simulink model "duffingSystem"  (R2020b)
settings: Solver=VariableStepAuto  StartTime=0.0  StopTime=60  RelTol=1e-8
values from neighbouring files (symbols this model uses):
  flag = 1    [aae666_hw4_p4.m]
  k1 = 1.25    [aae666_hw4_p4.m]
  k2 = 1.5    [aae666_hw4_p4.m]
settings Model: Creator=Tomo  LastModifiedBy=Tomo

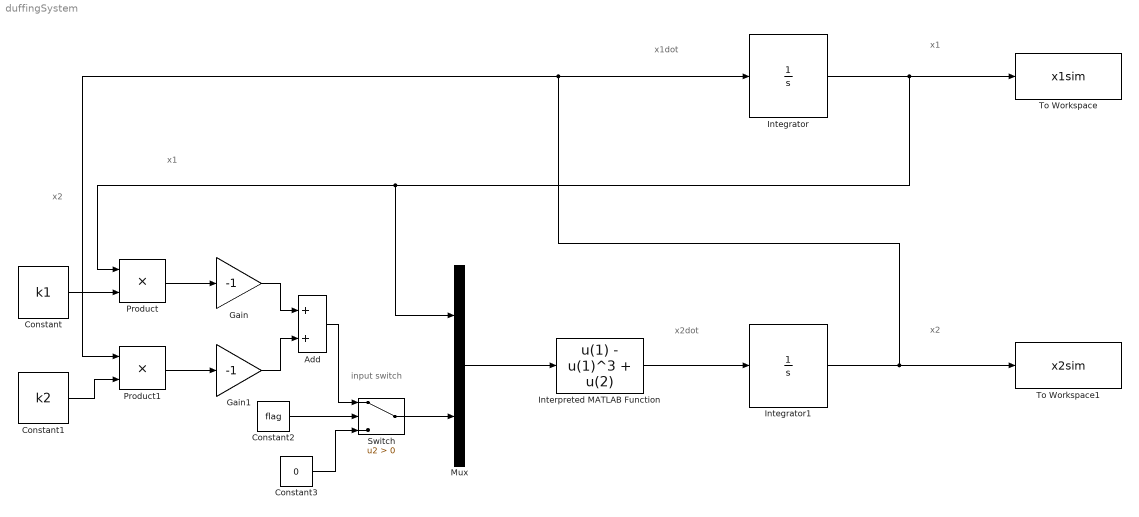
== system duffingSystem ==
  note: input switch
  note: x1dot
  note: x2dot
  note: x1
  note: x2
  note: x1
  note: x2
  Add : Sum
  Constant : Constant  Value=k1
  Constant1 : Constant  Value=k2
  Constant2 : Constant  Value=flag
  Constant3 : Constant  Value=0
  Gain : Gain  Gain=-1
  Gain1 : Gain  Gain=-1
  Integrator : Integrator
  Integrator1 : Integrator
  Interpreted MATLAB Function : MATLABFcn  MATLABFcn=u(1) - u(1)^3 + u(2)
  Mux : Mux  Inputs=2
  Product : Product
  Product1 : Product
  Switch : Switch  Criteria=u2 > Threshold
  To Workspace : ToWorkspace  VariableName=x1sim  SaveFormat=Structure With Time  SampleTime=-1
  To Workspace1 : ToWorkspace  VariableName=x2sim  SaveFormat=Structure With Time  SampleTime=-1
  wires:
  Integrator1/1 -> To Workspace1/1, Product1/1, Integrator/1
  Integrator/1 -> Product/1, Mux/1, To Workspace/1
  Mux/1 -> Interpreted MATLAB Function/1
  Interpreted MATLAB Function/1 -> Integrator1/1
  Constant/1 -> Product/2
  Constant1/1 -> Product1/2
  Product1/1 -> Gain1/1
  Product/1 -> Gain/1
  Gain/1 -> Add/1
  Gain1/1 -> Add/2
  Constant2/1 -> Switch/2
  Add/1 -> Switch/1
  Constant3/1 -> Switch/3
  Switch/1 -> Mux/2
